simulink model "PD_gravita2015"  (R2017b)
settings: Solver=FixedStepAuto  StartTime=0.0  StopTime=tf  FixedStep=T  RelTol=1e-3
values from neighbouring files (symbols this model uses):
  Kd = 300*[1;1;1;1;1;1]    [PDpiuGravita.m]    (also in dinamica_inversa.m = diag([2*zita(1)*w_n(1) 2*zita(2)*w_n(2) 2*zita(3)*w_n(3) 2*z; mainPD.m = 500*ones(6,1))
  Kp = diag([500 500 500 50])    [Approccio1.m]    (also in Approccio2.m = 10*diag([50 50 50 5]); Approccio3.m = 10*diag([50 50 50 5]); InversioneCinematica.m = diag([100 100 10 10]); PDpiuGravita.m = 1200*[1;1;1;1;1;1])
undefined symbols (not defined in the file or in its folder): DirectDynamicsSim, Gravity
settings Model: Creator=Giovanni  LastModifiedBy=Giovanni
settings OptimizationCC: LifeSpan=inf
settings DebuggingCC: SFExecutionAtInitializationDiag=none
settings CodeAppCC: StateflowObjectComments=on

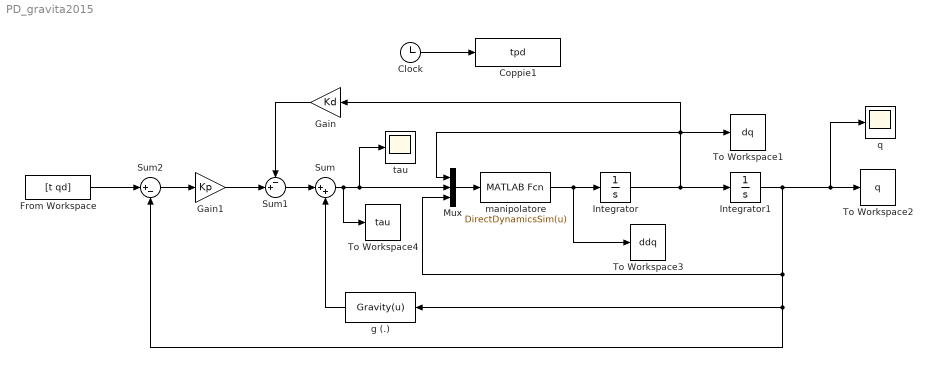
== system PD_gravita2015 ==
  Clock : Clock
  Coppie1 : ToWorkspace  VariableName=tpd  SampleTime=-1
  From Workspace : FromWorkspace  VariableName=[t qd]  SampleTime=0
  Gain : Gain  Gain=Kd
  Gain1 : Gain  Gain=Kp
  Integrator : Integrator  InitialCondition=zeros(6,1)
  Integrator1 : Integrator  InitialCondition=zeros(6,1)
  Mux : Mux  Inputs=3
  Sum : Sum  Inputs=|++
  Sum1 : Sum  Inputs=-+|
  Sum2 : Sum  Inputs=|+-
  To Workspace1 : ToWorkspace  VariableName=dq  SampleTime=-1
  To Workspace2 : ToWorkspace  VariableName=q  SampleTime=-1
  To Workspace3 : ToWorkspace  VariableName=ddq  SampleTime=-1
  To Workspace4 : ToWorkspace  VariableName=tau  SampleTime=-1
  g (.) : MATLABFcn  MATLABFcn=Gravity(u)
  manipolatore : MATLABFcn  MATLABFcn=DirectDynamicsSim(u)
  q : Scope
  "tau " : Scope
  wires:
  Clock/1 -> Coppie1/1
  manipolatore/1 -> To Workspace3/1, Integrator/1
  Integrator1/1 -> q/1, To Workspace2/1, Sum2/2, g (.)/1, Mux/3
  Integrator/1 -> Integrator1/1, Gain/1, Mux/1, To Workspace1/1
  Mux/1 -> manipolatore/1
  Sum/1 -> To Workspace4/1, "tau "/1, Mux/2
  g (.)/1 -> Sum/2
  Sum1/1 -> Sum/1
  Gain/1 -> Sum1/1
  Gain1/1 -> Sum1/2
  Sum2/1 -> Gain1/1
  From Workspace/1 -> Sum2/1
